simulink model "CruiseControl_pp"  (R2015b)
settings: Solver=ode3  StartTime=0.0  StopTime=16  FixedStep=0.1  RelTol=1e-3
PreLoadFcn:
  | CruiseControl_dd;
libraries: propertyLib x2, ctrlVerLib x1
settings Model: SnapshotInterval=1  Creator=The MathWorks Inc.  LastModifiedBy=colosky
settings DataIOCC: SaveFormat=Array  SaveOutput=off  SaveTime=off
settings OptimizationCC: DefaultParameterBehavior=Inlined  InlineInvariantSignals=on  ExpressionDepthLimit=2147483647  InitFltsAndDblsToZero=on
settings DebuggingCC: SaveWithParameterizedLinksMsg=none  UnderspecifiedInitializationDetection=Classic  MergeDetectMultiDrivingBlocksExec=none  SolverPrmCheckMsg=warning  FcnCallInpInsideContextMsg=UseLocalSettings  StateNameClashWarn=warning  StrictBusMsg=ErrorOnBusTreatedAsVector
settings HardwareCC: ProdBitPerPointer=32  ProdLargestAtomicFloat=None  ProdIntDivRoundTo=Undefined  ProdEndianess=Unspecified  ProdWordSize=32  ProdHWDeviceType=32-bit Generic
settings SFSimCC: SimParseCustomCode=off
settings GRTTargetCC: TargetFcnLib=ansi_tfl_tmw.mat  GeneratePreprocessorConditionals=Disable all  CombineOutputUpdateFcns=off  GRTInterface=on
settings ConfigComp: RecordCoverage=on  CovMetricSettings=dcme  CovHtmlReporting=off  CovSaveCumulativeToWorkspaceVar=off  CovSaveSingleToWorkspaceVar=off  CovModelRefEnable=Off  CovSFcnEnable=off  DVMode=PropertyProving  DVMaxProcessTime=3000  DVDisplayUnsatisfiableObjectives=on  DVAutomaticStubbing=off  DVMakeOutputFilesUnique=off  DVParameters=on  DVParametersUseConfig=on  DVModelCoverageObjectives=MCDC  DVMaxTestCaseSteps=500  DVTestSuiteOptimization=CombinedObjectives  DVAssertions=EnableAll  DVProofAssumptions=EnableAll  DVDetectIntegerOverflow=off  DVDetectActiveLogic=on  DVMaxViolationSteps=10  DVSaveDataFile=off  DVReportIncludeGraphics=on  DVDisplayResultsOnModel=on

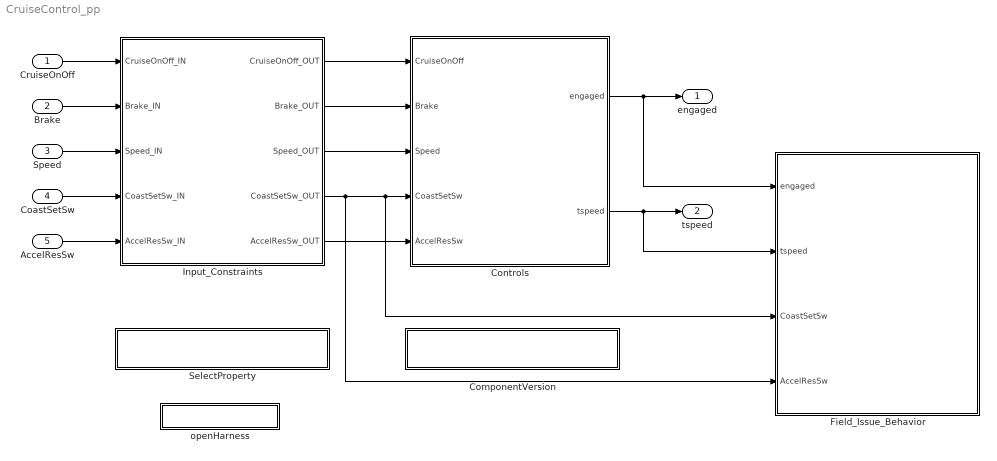
== system CruiseControl_pp ==
  CruiseOnOff : Inport  OutDataTypeStr=boolean  PortDimensions=1
  Brake : Inport  Port=2  OutDataTypeStr=boolean  PortDimensions=1
  Speed : Inport  Port=3  OutDataTypeStr=uint8  PortDimensions=1
  CoastSetSw : Inport  Port=4  OutDataTypeStr=boolean  PortDimensions=1
  AccelResSw : Inport  Port=5  OutDataTypeStr=boolean  PortDimensions=1
  ComponentVersion : Subsystem  mask(ControlsVersion){compVer=Execution Order Fix}
      mask help: Selects the block choice for the "Controls" subystem.
      mask init:
      | compVer = get_param(gcb,'compVer');
      | compBlk = find_system(bdroot,'LookUnderMasks','on','regexp','on',...
      |     'TemplateBlock','\w+','Name','^Controls$');
      | 
      | compBlk = compBlk{1};
      | if isempty(compBlk)
      |     disp('SelectProperty:  Error! Unable to find "Controls" configurable subsystem');
      |     return;
      | end
      | switch (compVer)
      |     case 'Original'
      |         set_param(compBlk,'BlockChoice','CtrlA_Original');
      |     case 'Sneak Fix'
      |         set_param(compBlk,'BlockChoice','CtrlB_Sneak_fix');
      |     case 'Execution Order Fix'
      |         set_param(compBlk,'BlockChoice','CtrlC_ExecOrder_fix');
      |     case 'Execution Order Sneak Fix'
      |         set_param(compBlk,'BlockChoice','CtrlD_ExecOrderSneak_fix');
      |     case 'Execution Order Sneak Double Reject Fix'
      |         set_param(compBlk,'BlockChoice','CtrlE_ExecOrderSneakDblReject_fix');
      |     case 'Execution Order Limit Check Fix'
      |         set_param(compBlk,'BlockChoice','CtrlF_ExecOrderLimCheck_fix');
      |     case 'Execution Order Limit Check Sneak Fix'
      |         set_param(compBlk,'BlockChoice','CtrlG_ExecOrderLimCheckSneak_fix');
      |     case 'All Fix'
      |         set_param(compBlk,'BlockChoice','CtrlH_All_fix');
      | end
      mask TypeOptions compVer: Original | Sneak Fix | Execution Order Fix | Execution Order Sneak Fix | Execution Order Sneak Double Reject Fix | Execution Order Limit Check Fix | Execution Order Limit Check Sneak Fix | All Fix
      mask DialogControl oprnCompLib Prompt: Open Component Lib
      mask DialogControl oprnCompLib Callback:
      | close_system('ctrlVerLib');
      | open_system('ctrlVerLib');
      mask Display: disp(['Selected Version to Verify:' char(10) get_param(gcb,'compVer')]);
  Controls : Subsystem  BlockChoice=CtrlC_ExecOrder_fix
      settings: AttributesFormatString=%<BlockChoice>  TemplateBlock=ctrlVerLib/ControlsCfgSub  MemberBlocks=CtrlA_Original,CtrlB_Sneak_fix,CtrlC_ExecOrder_fix,CtrlD_ExecOrderSneak_fix,CtrlE_ExecOrderSneakDblReject_fix,CtrlF_ExecOrderLimCheck_fix,CtrlG_ExecOrderLimCheckSneak_fix,CtrlH_All_fix
  Field_Issue_Behavior : Subsystem  BlockChoice=Prop_coast_pulse
      link override Prop_accel_overspeed/Compare To Constant: const=92
      link override Prop_tspeed_LE_90/Compare To Constant: const=90
      settings: AttributesFormatString=%<BlockChoice>  TemplateBlock=propertyLib/PropertyCfgSub  MemberBlocks=Prop_accel_overspeed,Prop_coast,Prop_coast_minspeed,Prop_coast_pulse,Prop_coast_pulse_eml,Prop_none,Prop_tspeed_LE_90
  Input_Constraints : Subsystem  BlockChoice=Assum_coast_pulse
      settings: AttributesFormatString=%<BlockChoice>  TemplateBlock=propertyLib/AssumptionCfgSub  MemberBlocks=Assum_accel_overspeed,Assum_coast,Assum_coast_minspeed,Assum_coast_pulse,Assum_coast_pulse_eml,Assum_none,Assum_tspeed_LE_90
  SelectProperty : Subsystem  mask(PropertySelection){property2prove=CoastSet pulse with tspeed decrease}
      mask help: Selects the block choice for the "Input_Constraints" and "Field_Issue_Behavior" subystems.
      mask init:
      | prop = get_param(gcb,'property2prove');
      | assumpBlk = find_system(bdroot,'LookUnderMasks','on','regexp','on',...
      |     'TemplateBlock','\w+','Name',...
      |     '^Input_Constraints$');
      | %    '^Assumption');
      | 
      | assumpBlk = assumpBlk{1};
      | propBlk = find_system(bdroot,'LookUnderMasks','on','regexp','on',...
      |     'TemplateBlock','\w+','Name',...
      |     '^Field_Issue_Behavior$');
      | %    '^Property');
      |     
      | 
      | propBlk = propBlk{1};
      | if isempty(assumpBlk) || isempty(propBlk)
      |     disp('SelectProperty:  Error! Unable to find configurable subsystems');
      |     return;
      | end
      | switch (prop)
      |     case 'None'
      |         set_param(assumpBlk,'BlockChoice','Assum_none');
      |         set_param(propBlk,'BlockChoice','Prop_none');
      |     case 'tspeed<=90'
      |         set_param(assumpBlk,'BlockChoice','Assum_tspeed_LE_90');
      |         set_param(propBlk,'BlockChoice','Prop_tspeed_LE_90');
      |     case 'CoastSet with tspeed decrease'
      |         set_param(assumpBlk,'BlockChoice','Assum_coast');
      |         set_param(propBlk,'BlockChoice','Prop_coast');
      |     case 'CoastSet pulse with tspeed decrease'     
      |         set_param(assumpBlk,'BlockChoice','Assum_coast_pulse');
      |         set_param(propBlk,'BlockChoice','Prop_coast_pulse');
      |     case 'CoastSet pulse (eml) with tspeed decrease'     
      |         set_param(assumpBlk,'BlockChoice','Assum_coast_pulse_eml');
      |         set_param(propBlk,'BlockChoice','Prop_coast_pulse_eml');
      |     case 'CoastSet with tspeed limit decrease'
      |         set_param(assumpBlk,'BlockChoice','Assum_coast_minspeed');
      |         set_param(propBlk,'BlockChoice','Prop_coast_minspeed');
      |     case 'Accel overspeed'
      |         set_param(assumpBlk,'BlockChoice','Assum_accel_overspeed');
      |         set_param(propBlk,'BlockChoice','Prop_accel_overspeed');
      |     otherwise
      |         disp('SelectProperty:  Error! Unable to find configurable subsystems');
      | end
      mask TypeOptions property2prove: None | tspeed<=90 | CoastSet with tspeed decrease | CoastSet pulse with tspeed decrease | CoastSet pulse (eml) with tspeed decrease | CoastSet with tspeed limit decrease | Accel overspeed
      mask DialogControl openPropLib Prompt: Open Prop Lib
      mask DialogControl openPropLib Callback:
      | close_system('propertyLib');
      | open_system('propertyLib');
      mask Display: disp(['Selected Property to Prove:' char(10) get_param(gcb,'property2prove')]);
  openHarness : Subsystem
      settings: OpenFcn=|
      | switch (get_param([bdroot '/ComponentVersion'],'compVer'))
      | case 'Execution Order Fix'
      |     load_PP_harness_FieldIssue;
      | case 'Execution Order Sneak Fix'
      |     load_PP_harness_ReqProve;
      | case 'Execution Order Sneak Double Reject Fix'
      |     load_PP_harness_ReqWithParsProve
      | end
      mask Display: disp(['Open Harness']);
  engaged : Outport  OutDataTypeStr=boolean  PortDimensions=1
  tspeed : Outport  Port=2  OutDataTypeStr=uint8  PortDimensions=1
  wires:
  Controls/2(tspeed) -> Field_Issue_Behavior/2(tspeed), tspeed/1
  Controls/1(engaged) -> Field_Issue_Behavior/1(engaged), engaged/1
  AccelResSw/1 -> Input_Constraints/5(AccelResSw_IN)
  Speed/1 -> Input_Constraints/3(Speed_IN)
  CruiseOnOff/1 -> Input_Constraints/1(CruiseOnOff_IN)
  Brake/1 -> Input_Constraints/2(Brake_IN)
  CoastSetSw/1 -> Input_Constraints/4(CoastSetSw_IN)
  Input_Constraints/1(CruiseOnOff_OUT) -> Controls/1(CruiseOnOff)
  Input_Constraints/2(Brake_OUT) -> Controls/2(Brake)
  Input_Constraints/3(Speed_OUT) -> Controls/3(Speed)
  Input_Constraints/4(CoastSetSw_OUT) -> Field_Issue_Behavior/4(AccelResSw), Field_Issue_Behavior/3(CoastSetSw), Controls/4(CoastSetSw)
  Input_Constraints/5(AccelResSw_OUT) -> Controls/5(AccelResSw)

== system CruiseControl_pp/ComponentVersion ==

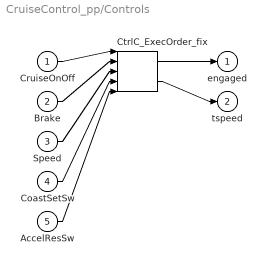
== system CruiseControl_pp/Controls ==
  CruiseOnOff : Inport
  Brake : Inport  Port=2
  Speed : Inport  Port=3
  CoastSetSw : Inport  Port=4
  AccelResSw : Inport  Port=5
  CtrlC_ExecOrder_fix : ctrlVerLib/CtrlC_ExecOrder_fix
  engaged : Outport
  tspeed : Outport  Port=2
  wires:
  CruiseOnOff/1 -> CtrlC_ExecOrder_fix/1
  Brake/1 -> CtrlC_ExecOrder_fix/2
  Speed/1 -> CtrlC_ExecOrder_fix/3
  CoastSetSw/1 -> CtrlC_ExecOrder_fix/4
  AccelResSw/1 -> CtrlC_ExecOrder_fix/5
  CtrlC_ExecOrder_fix/1 -> engaged/1
  CtrlC_ExecOrder_fix/2 -> tspeed/1

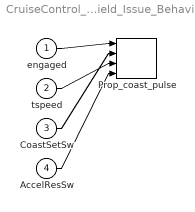
== system CruiseControl_pp/Field_Issue_Behavior ==
  engaged : Inport
  tspeed : Inport  Port=2
  CoastSetSw : Inport  Port=3
  AccelResSw : Inport  Port=4
  Prop_coast_pulse : propertyLib/Prop_coast_pulse
  wires:
  engaged/1 -> Prop_coast_pulse/1
  CoastSetSw/1 -> Prop_coast_pulse/2
  tspeed/1 -> Prop_coast_pulse/3
  AccelResSw/1 -> Prop_coast_pulse/4

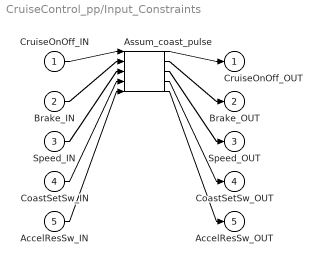
== system CruiseControl_pp/Input_Constraints ==
  CruiseOnOff_IN : Inport
  Brake_IN : Inport  Port=2
  Speed_IN : Inport  Port=3
  CoastSetSw_IN : Inport  Port=4
  AccelResSw_IN : Inport  Port=5
  Assum_coast_pulse : propertyLib/Assum_coast_pulse
  CruiseOnOff_OUT : Outport
  Brake_OUT : Outport  Port=2
  Speed_OUT : Outport  Port=3
  CoastSetSw_OUT : Outport  Port=4
  AccelResSw_OUT : Outport  Port=5
  wires:
  CruiseOnOff_IN/1 -> Assum_coast_pulse/1
  Brake_IN/1 -> Assum_coast_pulse/2
  Speed_IN/1 -> Assum_coast_pulse/3
  CoastSetSw_IN/1 -> Assum_coast_pulse/4
  AccelResSw_IN/1 -> Assum_coast_pulse/5
  Assum_coast_pulse/1 -> CruiseOnOff_OUT/1
  Assum_coast_pulse/2 -> Brake_OUT/1
  Assum_coast_pulse/3 -> Speed_OUT/1
  Assum_coast_pulse/4 -> CoastSetSw_OUT/1
  Assum_coast_pulse/5 -> AccelResSw_OUT/1

== system CruiseControl_pp/SelectProperty ==

== system CruiseControl_pp/openHarness ==
